simulink model "simulinkTutorial3"  (Simulink 7.7)
settings: Solver=ode45  StartTime=0.0  StopTime=40  RelTol=1e-3
settings Model: Creator=jiannianweng  LastModifiedBy=jiannianweng

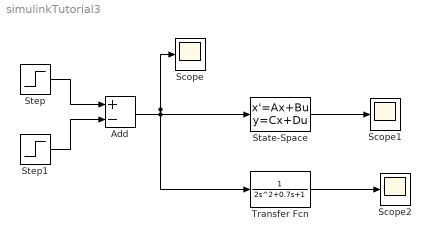
== system simulinkTutorial3 ==
  Add : Sum  Inputs=+-
  Scope : Scope
  Scope1 : Scope
  Scope2 : Scope
      settings: SaveName=ScopeData2
  State-Space : StateSpace  A=[-0.35 -0.5; 1 0]  B=[1;0]  C=[0 0.5]  D=0
  Step : Step  SampleTime=0
  Step1 : Step  Time=1.000000000001  SampleTime=0
  Transfer Fcn : TransferFcn  Denominator=[2 0.7 1]
  wires:
  Add/1 -> Scope/1, State-Space/1, Transfer Fcn/1
  Step/1 -> Add/1
  Step1/1 -> Add/2
  State-Space/1 -> Scope1/1
  Transfer Fcn/1 -> Scope2/1
